simulink model "Power2"  (Simulink 8.8)
settings: Solver=ode45  StartTime=0.0  StopTime=10.0  RelTol=1e-3  EnableMultiTasking=on
settings Model: SuppressorTable=22 serialization::archive 11 0 3 0 0 0 0 0  Creator=scaife  LastModifiedBy=hbourbou  ExtModeAutoUpdateStatusClock=off
settings DataIOCC: SignalLoggingName=sigsOut
settings OptimizationCC: LifeSpan=auto
settings DebuggingCC: SaveWithParameterizedLinksMsg=none  SignalResolutionControl=TryResolveAllWithWarning  MultiTaskDSMMsg=warning  MultiTaskCondExecSysMsg=none  FcnCallInpInsideContextMsg=error  StateNameClashWarn=none  SFUnexpectedBacktrackingDiag=error  SFNoUnconditionalDefaultTransitionDiag=error  SFExecutionAtInitializationDiag=warning
settings HardwareCC: TargetUnknown=on
settings SFSimCC: SimParseCustomCode=off
settings GRTTargetCC: GeneratePreprocessorConditionals=Use local settings

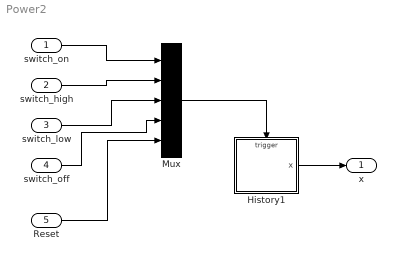
== system Power2 ==
  switch_on : Inport
  switch_high : Inport  Port=2
  switch_low : Inport  Port=3
  switch_off : Inport  Port=4
  Reset : Inport  Port=5
  History1 : Stateflow chart  TreatAsAtomicUnit=on
  Mux : Mux  Inputs=5
  x : Outport
  wires:
  switch_on/1 -> Mux/1
  Mux/1 -> History1/Trigger
  History1/1(x) -> x/1
  switch_high/1 -> Mux/2
  switch_low/1 -> Mux/3
  switch_off/1 -> Mux/4
  Reset/1 -> Mux/5

== stateflow chart History1 ==
  state Power_off
    en: x=0;
  state Power_on
    state Low/
      en: x=1;
    state High/
      en: x=2;
    Power_on -> (history) [order 1] : Reset
    (default) -> Low
    High -> Low : switch_high
    Low -> High : switch_low
  (default) -> Power_off
  Power_off -> Power_on : switch_on
  Power_on -> Power_off [order 1] : switch_off
  data: x output int32
  events: switch_on input EITHER_EDGE_EVENT; switch_off input EITHER_EDGE_EVENT; switch_high input RISING_EDGE_EVENT; switch_low input RISING_EDGE_EVENT; Reset input RISING_EDGE_EVENT
